simulink model "ANPC_Share"  (R2019b)
settings: Solver=ode23tb  StartTime=0.0  StopTime=n_ss_cycles/fout  RelTol=1e-3
values from neighbouring files (symbols this model uses):
  fout = 60    [FLEXINVETER_3LNPP_GF_Parameters_Rev06.m]
undefined symbols (not defined in the file or in its folder): fixed, plecs, Tinit, Twater
libraries: plecslib_extras x1
settings Model: Creator=graham.roberts  LastModifiedBy=105063423
settings DataIOCC: SaveFormat=Array  SignalLoggingSaveFormat=ModelDataLogs  ReturnWorkspaceOutputs=off
settings OptimizationCC: BlockReduction=off  BooleanDataType=off  ExpressionDepthLimit=2147483647  InitFltsAndDblsToZero=on  LifeSpan=inf
settings DebuggingCC: SaveWithParameterizedLinksMsg=none  UnderspecifiedInitializationDetection=Classic  MergeDetectMultiDrivingBlocksExec=none  SignalResolutionControl=TryResolveAllWithWarning  MultiTaskDSMMsg=warning  MultiTaskCondExecSysMsg=none  FcnCallInpInsideContextMsg=warning  StateNameClashWarn=warning  SFUnexpectedBacktrackingDiag=warning  SFNoUnconditionalDefaultTransitionDiag=warning  SFExecutionAtInitializationDiag=none  ArithmeticOperatorsInVariantConditions=warning
settings HardwareCC: ProdBitPerPointer=32  ProdBitPerSizeT=32  ProdBitPerPtrDiffT=32  ProdLargestAtomicFloat=None  ProdIntDivRoundTo=Undefined  ProdEndianess=Unspecified  ProdWordSize=32  ProdHWDeviceType=32-bit Generic  TargetUnknown=on
settings ModelReferenceCC: PropagateSignalLabelsOutOfModel=off
settings SFSimCC: SimUseLocalCustomCode=off  CustomCodeUndefinedFunction=UseInterfaceOnly
settings RTWCC: RTWUseLocalCustomCode=off
settings CodeAppCC: StateflowObjectComments=on
settings GRTTargetCC: TargetLangStandard=C89/C90 (ANSI)  GeneratePreprocessorConditionals=Disable all  CombineOutputUpdateFcns=off  GRTInterface=on
settings ConfigComp: CovMetricSettings=dw  CovHtmlReporting=on  CovSaveCumulativeToWorkspaceVar=on  CovSaveSingleToWorkspaceVar=on  CovExternalEMLEnable=off

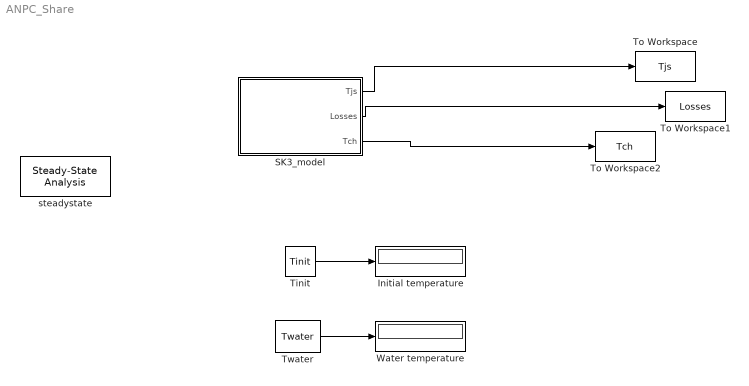
== system ANPC_Share ==
  Initial temperature : Display
  SK3_model : Subsystem  LoadFcn=plecs('sl', 200);  InitFcn=plecs('sl', 214);  StartFcn=plecs('sl', 208);  StopFcn=plecs('sl', 209);  mask(PlecsCircuit){PLECSData=<binary blob, 19804 chars, not shown>}
      mask prompts: PLECSData "PLECS Data (Do not delete or modify!)"
      mask init:
      | % PLACE CUSTOM INITIALIZATIONS ABOVE
      | % DO NOT REMOVE
      | plecs('sl', 215);
      | % DO NOT REMOVE
      settings: CopyFcn=plecs('sl', 203);  DeleteFcn=plecs('sl', 205);  UndoDeleteFcn=plecs('sl', 206);  PreSaveFcn=plecs('sl', 211);  PostSaveFcn=plecs('sl', 201);  NameChangeFcn=plecs('sl', 210);  DestroyFcn=plecs('sl', 207);  PreCopyFcn=plecs('sl', 216);  OpenFcn=plecs('sl', 202);  ErrorFcn=plerrorfcn
      mask Help: web(['file:///' fullfile(plecsdoc, 'creatingacircuit.html')])
      mask Display: disp('PLECS\nCircuit')
  Tinit : Constant  Value=Tinit
  To Workspace : ToWorkspace  VariableName=Tjs  SampleTime=-1
  To Workspace1 : ToWorkspace  VariableName=Losses  SampleTime=-1
  To Workspace2 : ToWorkspace  VariableName=Tch  SampleTime=-1
  Twater : Constant  Value=Twater
  Water temperature : Display
  steadystate : plecslib_extras/Analysis Tools/Steady-State Analysis  Period=fixed  TriggerType=rising  TimeSpan=1/fout  TStart=0  MaxIter=20  Tolerance=1e-6  Display=iteration  HideScopes=off  HiddenStates=error  FinalStateName=xSteadyState  NCycles=n_ss_cycles  JPert=1e-4  JacobianCalculation=fast  NInitCycles=0
  wires:
  Tinit/1 -> Initial temperature/1
  Twater/1 -> Water temperature/1
  SK3_model/2(Losses) -> To Workspace1/1
  SK3_model/1(Tjs) -> To Workspace/1
  SK3_model/3(Tch) -> To Workspace2/1

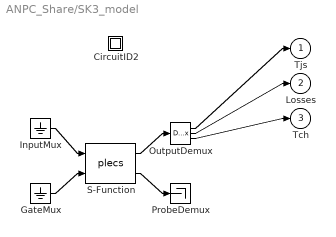
== system ANPC_Share/SK3_model ==
  " CircuitID2 " : Subsystem
  " GateMux " : Ground
  " InputMux " : Ground
  " OutputDemux " : Demux  Outputs=[ 6 12 3 ]
  " ProbeDemux " : Terminator
  " S-Function " : S-Function  FunctionName=plecs  SFunctionDeploymentMode=off  EnableBusSupport=off
  Tjs : Outport  PortDimensions=6
  Losses : Outport  Port=2  PortDimensions=12
  Tch : Outport  Port=3  PortDimensions=3
  wires:
  " InputMux "/1 -> " S-Function "/1
  " GateMux "/1 -> " S-Function "/2
  " S-Function "/1 -> " OutputDemux "/1
  " S-Function "/2 -> " ProbeDemux "/1
  " OutputDemux "/1 -> Tjs/1
  " OutputDemux "/2 -> Losses/1
  " OutputDemux "/3 -> Tch/1

== system ANPC_Share/SK3_model/ CircuitID2  ==
